simulink model "two_generators_motor"  (R2014a)
settings: Solver=ode23tb  StartTime=0.0  StopTime=0.1  FixedStep=Ts  MaxStep=1e-4  RelTol=1e-4
PreLoadFcn:
  | Ts=2.5e-5;
InitFcn:
  | Ts=2.5e-5;
libraries: powerlib x7
settings Model: Creator=gdudgeon  LastModifiedBy=cosorio
settings DataIOCC: SignalLoggingSaveFormat=ModelDataLogs
settings OptimizationCC: ExpressionDepthLimit=2147483647  InitFltsAndDblsToZero=on
settings DebuggingCC: SaveWithParameterizedLinksMsg=none  UnderspecifiedInitializationDetection=Classic  SignalResolutionControl=TryResolveAllWithWarning  MultiTaskDSMMsg=warning  MultiTaskCondExecSysMsg=none  FcnCallInpInsideContextMsg=UseLocalSettings  StateNameClashWarn=warning
settings RTWCC: IncludeERTFirstTime=on
settings GRTTargetCC: TargetFcnLib=ansi_tfl_tmw.mat  CombineOutputUpdateFcns=off  GRTInterface=on

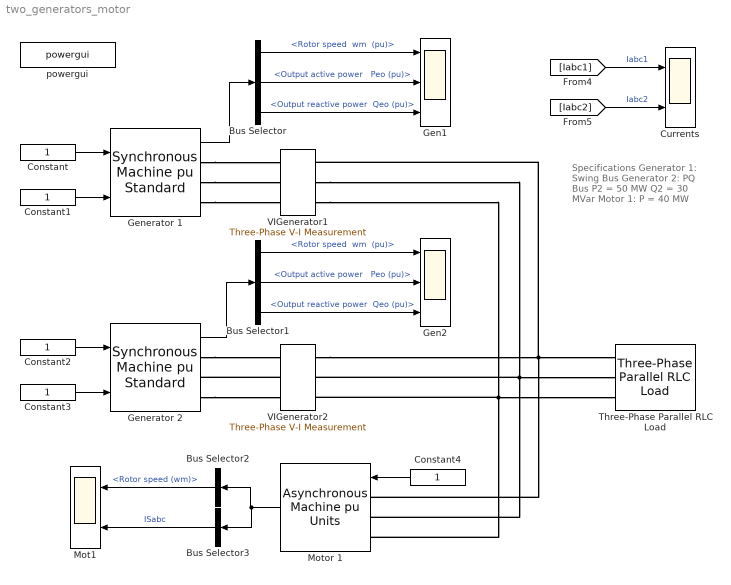
== system two_generators_motor ==
  note: Specifications
      | Generator 1:
      | Swing Bus
      | Generator 2:
      | PQ Bus
      | P2 = 50 MW
      | Q2 = 30 MVar
      | Motor 1:
      | P = 40 MW
  Bus Selector : BusSelector  OutputSignals="Mechanical.Rotor speed  wm  (pu),Output active power   Peo (pu),Output reactive power  Qeo (pu)"
  Bus Selector1 : BusSelector  OutputSignals="Mechanical.Rotor speed  wm  (pu),Output active power   Peo (pu),Output reactive power  Qeo (pu)"
  Bus Selector2 : BusSelector  OutputSignals=Mechanical.Rotor speed (wm)
  Bus Selector3 : BusSelector  OutputSignals=Stator measurements.Stator current is_a (pu),Stator measurements.Stator current is_b (pu),Stator measurements.Stator current is_c (pu)  OutputAsBus=on
  Constant{,1..4} (5 alike) : Constant
  Currents : Scope  NumInputPorts=2
      settings: YMin=-10000~-10000  YMax=10000~10000
  Gen1 : Scope  NumInputPorts=3
      settings: YMin=0~0~0  YMax=1.5~1~1  SaveName=ScopeData5
  Gen2 : Scope  NumInputPorts=3
      settings: YMin=0~0~0  YMax=1.5~1~1
  Generator 1 : powerlib/Machines/Synchronous Machine pu Standard  PresetModel=No  MechanicalLoad=Mechanical power Pm  ShowDetailedParameters=on  RotorType=Salient-pole  Units=per unit standard parameters  MeasurementBus=off  NominalParameters="[ 187E6  13800   60]"  Reactances1=[ 1.81, 0.3, 0.23, 1.76, 0.65, 0.25, 0.15 ]  Reactances2="[ 1.305, 0.296, 0.252, 0.474,  0.243,  0.18 ]"  dAxisTimeConstants=Open-circuit  qAxisTimeConstants=Short-circuit  TimeConstants1="[ 4.4849  0.0681  0.1  ]"  TimeConstants2=[ 8.0, 0.03, 1.0, 0.07 ]  TimeConstants3="[  4.49  0.0681  0.0513  ]"  TimeConstants4=[ 8.0, 0.03, 0.3371, 0.0295 ]  TimeConstants5=[ 1.01, 0.053, 0.1 ]  TimeConstants6=[ 1.3201, 0.023, 1.0, 0.07 ]  TimeConstants7=[0.012 0.003 0.003]  TimeConstants8=[ 1.3201, 0.0231, 0.3371, 0.0295 ]  StatorResistance=0.003  Mechanical="[ 3.7 0  20 ]"  PolePairs=20  InitialConditions="[ 0  0  0  0  0  0  0  0  1 ]"  SetSaturation=off  Saturation=[0.6404,0.7127,0.8441,0.9214,0.9956,1.082,1.19,1.316,1.457;0.7,0.7698,0.8872,0.9466,0.9969,1.046,1.1,1.151,1.201]  LoadFlowParameters=[2 70000000 0 0 30000000]  TsPowergui=0  TsBlock=-1  IterativeModel=Forward Euler  BusType=swing  Pref=0  Qref=0  Qmin=-inf  Qmax=inf  PLF=0  QLF=0
      settings: AttributesFormatString=%<NominalParameters>
  Generator 2 : powerlib/Machines/Synchronous Machine pu Standard  PresetModel=No  MechanicalLoad=Mechanical power Pm  ShowDetailedParameters=on  RotorType=Salient-pole  Units=per unit standard parameters  MeasurementBus=off  NominalParameters="[ 187E6  13800   60]"  Reactances1=[ 1.81, 0.3, 0.23, 1.76, 0.65, 0.25, 0.15 ]  Reactances2="[ 1.305, 0.296, 0.252, 0.474,  0.243,  0.18 ]"  dAxisTimeConstants=Open-circuit  qAxisTimeConstants=Short-circuit  TimeConstants1="[ 4.4849  0.0681  0.1  ]"  TimeConstants2=[ 8.0, 0.03, 1.0, 0.07 ]  TimeConstants3="[  4.49  0.0681  0.0513  ]"  TimeConstants4=[ 8.0, 0.03, 0.3371, 0.0295 ]  TimeConstants5=[ 1.01, 0.053, 0.1 ]  TimeConstants6=[ 1.3201, 0.023, 1.0, 0.07 ]  TimeConstants7=[0.012 0.003 0.003]  TimeConstants8=[ 1.3201, 0.0231, 0.3371, 0.0295 ]  StatorResistance=0.003  Mechanical="[ 3.7 0  20 ]"  PolePairs=20  InitialConditions="[ 0  0  0  0  0  0  0  0  1 ]"  SetSaturation=off  Saturation=[0.6404,0.7127,0.8441,0.9214,0.9956,1.082,1.19,1.316,1.457;0.7,0.7698,0.8872,0.9466,0.9969,1.046,1.1,1.151,1.201]  LoadFlowParameters=[4 50000000 0 0 30000000]  TsPowergui=0  TsBlock=-1  IterativeModel=Forward Euler  BusType=PQ  Pref=5e7  Qref=3e7  Qmin=-inf  Qmax=inf  PLF=0  QLF=0
      settings: AttributesFormatString=%<NominalParameters>
  Mot1 : Scope  NumInputPorts=2
      settings: YMin=0~-2  YMax=1.5~2  SaveName=ScopeData2
  Motor 1 : powerlib/Machines/Asynchronous Machine pu Units  PresetModel=No  MechanicalLoad=Torque Tm  ShowDetailedParameters=on  RotorType=Squirrel-cage  ReferenceFrame=Rotor  Units=pu  MeasurementBus=off  NominalParameters=[50e6 13800 60]  Stator=[0.01965 0.0397]  Rotor=[0.01909 0.0397]  Cage1=[0.01909 0.0397]  Cage2=[0.01909 0.0397]  Lm=1.354  Mechanical=[1 0.05479 2]  PolePairs=2  InitialConditions=[0 0 0 0 0 0 0 0]  SimulateSaturation=off  Saturation="[0.212,0.4201,0.8125,1.0979,1.4799,2.2457,3.2586,4.5763,6.4763 ;   0.5,0.7,0.9,1,1.1,1.2 ,1.3,1.4,1.5]"  LoadFlowParameters=40000000  TsPowergui=0  TsBlock=-1  IterativeModel=Forward Euler  Pmec=40e6
      settings: AttributesFormatString=%<NominalParameters>
  Three-Phase Parallel RLC Load : powerlib/Elements/Three-Phase Parallel RLC Load  LConnTagsString=A|B|C  Configuration=Y (grounded)  NominalVoltage=13800  NominalFrequency=60  ActivePower=120e6  InductivePower=70e6  CapacitivePower=100  Measurements=None  LoadType=constant Z
      settings: AttributesFormatString=|
      | Vn = %<NominalVoltage> Vrms
      | fn = %<NominalFrequency> Hz
      | P = %<ActivePower> W
      | QL = %<InductivePower> Var
      | QC = %<CapacitivePower> Var
  VIGenerator1 : powerlib/Measurements/Three-Phase V-I Measurement  VoltageMeasurement=no  SetLabelV=off  LabelV=Vabc  Vpu=off  VpuLL=off  CurrentMeasurement=yes  SetLabelI=on  LabelI=Iabc1  Ipu=off  Pbase=100e6  Vbase=500e3  OutputType=Complex  PhasorSimulation=off  PSBequivalent=0
  VIGenerator2 : powerlib/Measurements/Three-Phase V-I Measurement  VoltageMeasurement=no  SetLabelV=off  LabelV=Vabc  Vpu=off  VpuLL=off  CurrentMeasurement=yes  SetLabelI=on  LabelI=Iabc2  Ipu=off  Pbase=100e6  Vbase=500e3  OutputType=Complex  PhasorSimulation=off  PSBequivalent=0
  powergui : powerlib/powergui  Priority=2  SimulationMode=Continuous  SolverType=Tustin  SampleTime=Ts  frequency=60  SPID=off  DisableSnubberDevices=off  DisableRonSwitches=off  DisableVfSwitches=off  SwTol=0  Interpol=off  DisplayEquations=off  Ts=0  methode=off  frequencyindice=60  Pbase=100e6  ErrMax=1e-4  Iterations=50  UnitsV=kV  UnitsW=MW  FunctionMessages=off  echomessages=off  HookPort=off  EnableUseOfTLC=off  x0status=blocks  RestoreLinks=warning  ResistiveCurrentMeasurement=off  Frange=[0:2:500]  Ylog=off  Xlog=on  ShowGrid=off  save=off  variable=ZData  structure=Iabc2  ZoomFFT=on  StartTime=4  cycles=1  DisplayStyle=1  fundamental=60  FreqAxis=on  MaxFrequency=2000  frequencyindicesteady=1  RmsSteady=1  display=off
  wires:
  Constant/1 -> Generator 1/1
  Constant1/1 -> Generator 1/2
  Generator 1/1 -> Bus Selector/1
  Bus Selector/1 -> Gen1/1  "<Rotor speed  wm  (pu)>"
  Constant2/1 -> Generator 2/1
  Constant3/1 -> Generator 2/2
  Bus Selector1/1 -> Gen2/1  "<Rotor speed  wm  (pu)>"
  Generator 2/1 -> Bus Selector1/1
  [Iabc1] -> Currents/1  "Iabc1"
  [Iabc2] -> Currents/2  "Iabc2"
  Bus Selector1/2 -> Gen2/2  "<Output active power   Peo (pu)>"
  Bus Selector1/3 -> Gen2/3  "<Output reactive power  Qeo (pu)>"
  Bus Selector/2 -> Gen1/2  "<Output active power   Peo (pu)>"
  Bus Selector/3 -> Gen1/3  "<Output reactive power  Qeo (pu)>"
  Constant4/1 -> Motor 1/1
  Motor 1/1 -> Bus Selector3/1, Bus Selector2/1
  Bus Selector2/1 -> Mot1/1  "<Rotor speed (wm)>"
  Bus Selector3/1 -> Mot1/2  "ISabc"
  connections:
  Generator 1/RConn2 -- VIGenerator1/LConn2
  Generator 1/RConn1 -- VIGenerator1/LConn1
  Generator 1/RConn3 -- VIGenerator1/LConn3
  Generator 2/RConn1 -- VIGenerator2/LConn1
  VIGenerator2/LConn2 -- Generator 2/RConn2
  Generator 2/RConn3 -- VIGenerator2/LConn3
  VIGenerator2/RConn1 -- Motor 1/LConn1 -- VIGenerator1/RConn1 -- Three-Phase Parallel RLC Load/LConn1
  VIGenerator1/RConn2 -- Motor 1/LConn2 -- VIGenerator2/RConn2 -- Three-Phase Parallel RLC Load/LConn2
  VIGenerator1/RConn3 -- Motor 1/LConn3 -- VIGenerator2/RConn3 -- Three-Phase Parallel RLC Load/LConn3
